simulink model "RepCtrlScanner"  (R2018b)
settings: Solver=VariableStepAuto  StartTime=0.0  StopTime=10.0  RelTol=1e-3
values from neighbouring files (symbols this model uses):
  delayN1 = N-delayN2-nq    (= 152)    [ILCFF_NLIIC.m]    (also in ILCFF_ProgILC.m; ILCFF_ctrl.mat)
  delayN2 = delayK1    (= 47)    [ILCFF_NLIIC.m]    (also in ILCFF_ProgILC.m; ILCFF_ctrl.mat)
  Hz = 1/Ts    (= 20000)    [ILCFF_NLIIC.m]    (also in ILCFF_ProgILC.m; ILCFF_ctrl.mat)
  RefFreq = 400    [main.m]
  SinePulseAmp = 0    [main.m]
  TriPulseAmp = 5    [main.m]
  TriPulseT = 1/RefFreq    (= 0.0025)    [main.m]
  Ts = 0.00005    (= 5e-05)    [ILCFF_NLIIC.m]    (also in ILCFF_ProgILC.m; main.m = 1/Hz)
libraries: cstblocks x4, simulink x1
settings Model: Creator=NTU  LastModifiedBy=NTU

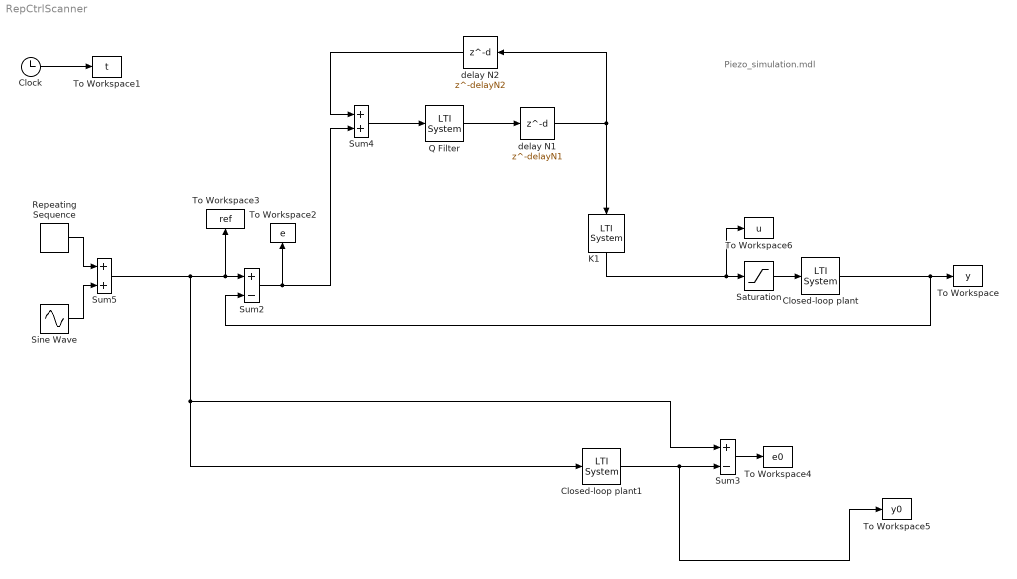
== system RepCtrlScanner ==
  note: Piezo_simulation.mdl
  Clock : Clock
  Closed-loop plant : cstblocks/LTI System  sys=P  IC=[]
  Closed-loop plant1 : cstblocks/LTI System  sys=P  IC=[]
  K1 : cstblocks/LTI System  sys=FF  IC=[]
  Q Filter : cstblocks/LTI System  sys=Q  IC=[]
  Repeating Sequence : simulink/Sources/Repeating Sequence  rep_seq_t=[0 TriPulseT/2 TriPulseT]  rep_seq_y=[TriPulseAmp -TriPulseAmp TriPulseAmp]
  Saturation : Saturate  UpperLimit=12.5  LowerLimit=-12.5
  Sine Wave : Sin  Amplitude=SinePulseAmp  Frequency=RefFreq*2*pi()  SampleTime=0
  Sum2 : Sum  Inputs=+-  SaturateOnIntegerOverflow=on  InputSameDT=on  OutDataTypeStr=Inherit: Same as first input
  Sum3 : Sum  Inputs=+-  SaturateOnIntegerOverflow=on  InputSameDT=on  OutDataTypeStr=Inherit: Same as first input
  Sum4 : Sum  SaturateOnIntegerOverflow=on  InputSameDT=on  OutDataTypeStr=Inherit: Same as first input
  Sum5 : Sum  SaturateOnIntegerOverflow=on  InputSameDT=on  OutDataTypeStr=Inherit: Same as first input
  To Workspace : ToWorkspace  VariableName=y  SampleTime=1/Hz
  To Workspace1 : ToWorkspace  VariableName=t  SampleTime=1/Hz
  To Workspace2 : ToWorkspace  VariableName=e  SampleTime=1/Hz
  To Workspace3 : ToWorkspace  VariableName=ref  SampleTime=1/Hz
  To Workspace4 : ToWorkspace  VariableName=e0  SampleTime=1/Hz
  To Workspace5 : ToWorkspace  VariableName=y0  SampleTime=1/Hz
  To Workspace6 : ToWorkspace  VariableName=u  SampleTime=1/Hz
  delay N1 : Delay  DelayLength=delayN1  InputProcessing=Inherited  SampleTime=Ts
  delay N2 : Delay  DelayLength=delayN2  InputProcessing=Inherited  SampleTime=Ts
  wires:
  Q Filter/1 -> delay N1/1
  K1/1 -> To Workspace6/1, Saturation/1
  Sum2/1 -> To Workspace2/1, Sum4/2
  Sine Wave/1 -> Sum5/2
  Sum3/1 -> To Workspace4/1
  Saturation/1 -> Closed-loop plant/1
  Clock/1 -> To Workspace1/1
  Sum4/1 -> Q Filter/1
  delay N1/1 -> K1/1, delay N2/1
  Repeating Sequence/1 -> Sum5/1
  delay N2/1 -> Sum4/1
  Closed-loop plant/1 -> Sum2/2, To Workspace/1
  Closed-loop plant1/1 -> To Workspace5/1, Sum3/2
  Sum5/1 -> Closed-loop plant1/1, Sum3/1, To Workspace3/1, Sum2/1
